simulink model "upsample_ref3"  (Simulink 4.00)
settings: Solver=FixedStepDiscrete  SolverMode=MultiTasking  StartTime=0.0  StopTime=30  RelTol=1e-3
PostLoadFcn:
  | set_param(gcs,'SimulationCommand','Update')
libraries: dspsrcs3 x1, dspsigops x1
settings Model: RequirementInfo=9  Creator=ckamachi  LastModifiedBy=ckamachi  LimitDataPoints=off  ExtModeTrigMode=oneshot  ExtModeArmWhenConnect=off  BlockReductionOpt=off

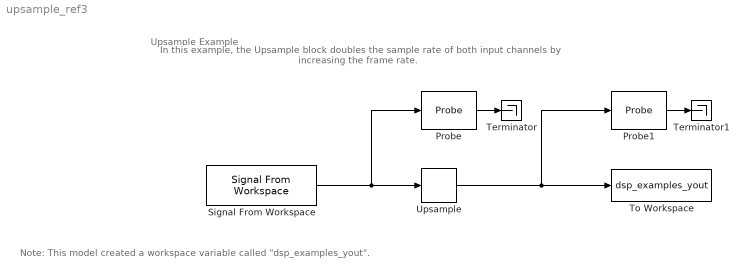
== system upsample_ref3 ==
  note: Upsample Example
  note: In this example, the Upsample block doubles the sample rate
      | of both input channels by increasing the frame rate.
  note: Note: This model created a workspace variable called "dsp_examples_yout".
  Probe : Probe  ProbeWidth=off  ProbeSampleTime=on  ProbeComplexSignal=off  ProbeSignalDimensions=off
  Probe1 : Probe  ProbeWidth=off  ProbeSampleTime=on  ProbeComplexSignal=off  ProbeSignalDimensions=off
  Signal From Workspace : dspsrcs3/Signal From Workspace  X=[(1:100)' (-1:-1:-100)']  Ts=0.25  nsamps=4  OutputAfterFinalValue=Setting To Zero
  Terminator : Terminator
  Terminator1 : Terminator
  To Workspace : ToWorkspace  VariableName=dsp_examples_yout  SampleTime=-1  SaveFormat=Array
  Upsample : dspsigops/Upsample  N=2  phase=0  ic=0  mode=Maintain input frame size
  wires:
  Upsample/1 -> To Workspace/1, Probe1/1
  Signal From Workspace/1 -> Probe/1, Upsample/1
  Probe/1 -> Terminator/1
  Probe1/1 -> Terminator1/1
